simulink model "Full_system_3DOF"  (R2015b)
settings: Solver=ode45  StartTime=0.0  StopTime=55  FixedStep=0.0001  RelTol=eps
values from neighbouring files (symbols this model uses):
  All_Inertia = 1e-9*[177248429.51 3410266.03 17326.3 ... (first row only)    [init_sim_3DOF.m]    (also in init_sim_4DOF.m)
  B_m = 0.5*8815e-4    (= 0.44075)    [init_sim_3DOF.m]
  c_B = 0    [init_sim_1DOF.m]    (also in init_sim_4DOF.m)
  c_flux = 1    [init_sim_3DOF.m]
  c_G = 0.5    [init_sim_3DOF.m]    (also in init_sim_4DOF.m = 0)
  c_trans = c_G    (= 0.5)    [init_sim_3DOF.m]    (also in init_sim_4DOF.m = 0)
  Float_CoM = CoM-N_DCM_G*G_r_CB    [init_sim_3DOF.m]    (also in init_sim_4DOF.m = CoM+N_DCM_G*G_r_CB)
  Float_init_vel = OS_init_vel    [init_sim_3DOF.m]    (also in init_sim_4DOF.m)
  OS_init_omega = 0    [init_sim_1DOF.m]    (also in init_sim_3DOF.m; init_sim_4DOF.m = [0 0 0]'; init_sim_6DOF.m = [0 0 0]')
  OS_rotation = 0    [init_sim_1DOF.m]    (also in init_sim_3DOF.m; init_sim_4DOF.m = [0 0 0]'; init_sim_6DOF.m = [0 0 0]')
  SROA_Inertia = 1e7*eye(3)    [init_sim_3DOF.m]    (also in init_sim_4DOF.m)
  SROA_Mass = 100000    [init_sim_3DOF.m]    (also in init_sim_4DOF.m)
  V = [0 0 0 0 0 0]'    [init_sim_1DOF.m]    (also in init_sim_3DOF.m; init_sim_4DOF.m; init_sim_6DOF.m)
  Whole_Mass = 12.38866    [init_sim_3DOF.m]    (also in init_sim_4DOF.m)
undefined symbols (not defined in the file or in its folder): EM_mu, EM_xyz, origin, OS_mu_0, OS_xyz_0
libraries: my_ACS_library x1
settings Model: Creator=user  LastModifiedBy=user
settings DataIOCC: SaveFormat=Array
settings DebuggingCC: SolverPrmCheckMsg=warning
settings HardwareCC: ProdBitPerPointer=32  ProdLargestAtomicFloat=None  ProdIntDivRoundTo=Undefined  ProdEndianess=Unspecified  ProdWordSize=32  ProdHWDeviceType=32-bit Generic
settings GRTTargetCC: GeneratePreprocessorConditionals=Disable all
settings ConfigComp: CovModelRefEnable=Off  CovSFcnEnable=off

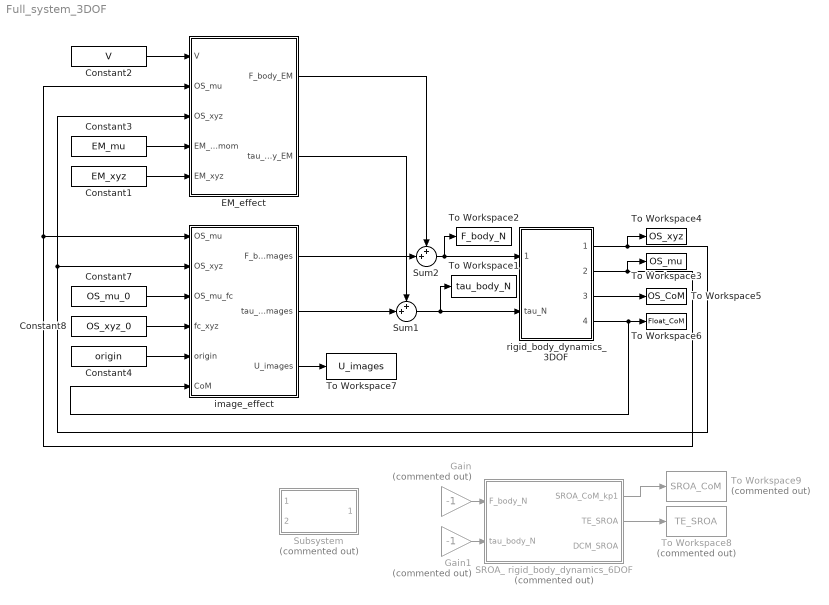
== system Full_system_3DOF ==
  Constant1 : Constant  Value=EM_xyz
  Constant2 : Constant  Value=V
  Constant3 : Constant  Value=EM_mu
  Constant4 : Constant  Value=origin
  Constant7 : Constant  Value=OS_mu_0  VectorParams1D=off
  Constant8 : Constant  Value=OS_xyz_0
  EM_effect : MATLAB Function  TreatAsAtomicUnit=on
  Gain : Gain  Commented=on  Gain=-1
  Gain1 : Gain  Commented=on  Gain=-1
  SROA_ rigid_body_dynamics_6DOF : Subsystem  Commented=on
  Subsystem : Subsystem  Commented=on
  Sum1 : Sum  Inputs=++|
  Sum2 : Sum  Inputs=++|
  To Workspace1 : ToWorkspace  VariableName=tau_body_N  SaveFormat=Timeseries  SampleTime=-1
  To Workspace2 : ToWorkspace  VariableName=F_body_N  SaveFormat=Timeseries  SampleTime=-1
  To Workspace3 : ToWorkspace  VariableName=OS_mu  SaveFormat=Timeseries  SampleTime=-1
  To Workspace4 : ToWorkspace  VariableName=OS_xyz  SaveFormat=Timeseries  SampleTime=-1
  To Workspace5 : ToWorkspace  VariableName=OS_CoM  SaveFormat=Timeseries  SampleTime=-1
  To Workspace6 : ToWorkspace  VariableName=Float_CoM  SaveFormat=Timeseries  SampleTime=-1
  To Workspace7 : ToWorkspace  VariableName=U_images  SaveFormat=Timeseries  SampleTime=-1
  To Workspace8 : ToWorkspace  Commented=on  VariableName=TE_SROA  SaveFormat=Timeseries  SampleTime=-1
  To Workspace9 : ToWorkspace  Commented=on  VariableName=SROA_CoM  SaveFormat=Timeseries  SampleTime=-1
  image_effect : MATLAB Function  TreatAsAtomicUnit=on
  rigid_body_dynamics_3DOF : Subsystem
  wires:
  Constant3/1 -> EM_effect/4(EM_magmom)
  Constant1/1 -> EM_effect/5(EM_xyz)
  image_effect/1(F_body_images) -> Sum2/2
  image_effect/2(tau_body_images) -> Sum1/2
  EM_effect/2(tau_body_EM) -> Sum1/1
  EM_effect/1(F_body_EM) -> Sum2/1
  image_effect/3(U_images) -> To Workspace7/1
  Sum2/1 -> To Workspace2/1, rigid_body_dynamics_3DOF/1(Force_N)
  Sum1/1 -> To Workspace1/1, rigid_body_dynamics_3DOF/2(tau_N)
  rigid_body_dynamics_3DOF/4(Float_CoM) -> image_effect/6(CoM), To Workspace6/1
  Constant2/1 -> EM_effect/1(V)
  rigid_body_dynamics_3DOF/1(OS_xyz) -> To Workspace4/1, EM_effect/3(OS_xyz), image_effect/2(OS_xyz)
  rigid_body_dynamics_3DOF/2(OS_mu) -> To Workspace3/1, EM_effect/2(OS_mu), image_effect/1(OS_mu)
  rigid_body_dynamics_3DOF/3(OS_CoM) -> To Workspace5/1
  Constant7/1 -> image_effect/3(OS_mu_fc)
  Constant8/1 -> image_effect/4(fc_xyz)
  Constant4/1 -> image_effect/5(origin)
  Gain/1 -> SROA_ rigid_body_dynamics_6DOF/1(F_body_N)
  Gain1/1 -> SROA_ rigid_body_dynamics_6DOF/2(tau_body_N)
  SROA_ rigid_body_dynamics_6DOF/2(TE_SROA) -> To Workspace8/1
  SROA_ rigid_body_dynamics_6DOF/1(SROA_CoM_kp1) -> To Workspace9/1

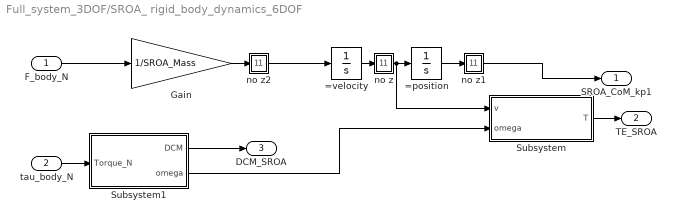
== system Full_system_3DOF/SROA_ rigid_body_dynamics_6DOF ==
  F_body_N : Inport
  tau_body_N : Inport  Port=2
  =position : Integrator  InitialCondition=[0 0 0]'
  =velocity : Integrator  InitialCondition=[0 0 0]'
  Gain : Gain  Gain=1/SROA_Mass
  Subsystem : Subsystem
  Subsystem1 : Subsystem
  no z : Subsystem
  no z1 : Subsystem
  no z2 : Subsystem
  SROA_CoM_kp1 : Outport
  TE_SROA : Outport  Port=2  PortDimensions=1
  DCM_SROA : Outport  Port=3  PortDimensions=[3 3]
  wires:
  Subsystem/1(T) -> TE_SROA/1
  F_body_N/1 -> Gain/1
  =velocity/1 -> no z/1(In1)
  no z/1(Out1) -> Subsystem/1(v), =position/1
  =position/1 -> no z1/1(In1)
  Gain/1 -> no z2/1(In1)
  no z2/1(Out1) -> =velocity/1
  no z1/1(Out1) -> SROA_CoM_kp1/1
  tau_body_N/1 -> Subsystem1/1(Torque_N)
  Subsystem1/2(omega) -> Subsystem/2(omega)
  Subsystem1/1(DCM) -> DCM_SROA/1

== system Full_system_3DOF/Subsystem ==
  SROA_CoM : Inport
  SROA_DCM : Inport  Port=2
  Constant2 : Constant  Value=origin
  MATLAB Function : MATLAB Function  TreatAsAtomicUnit=on
  SROA_origin : Outport
  wires:
  Constant2/1 -> MATLAB Function/1(origin)
  SROA_CoM/1 -> MATLAB Function/2(CoM)
  MATLAB Function/1(origin_new) -> SROA_origin/1
  SROA_DCM/1 -> MATLAB Function/3(DCM)

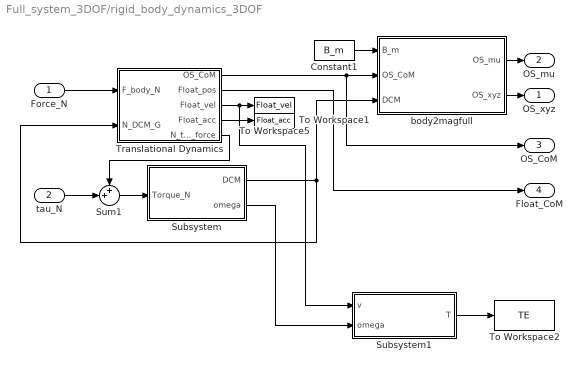
== system Full_system_3DOF/rigid_body_dynamics_3DOF ==
  Force_N : Inport
  tau_N : Inport  Port=2
  Constant1 : Constant  Value=B_m
  Subsystem : Subsystem
  Subsystem1 : Subsystem
  Sum1 : Sum  Inputs=++|
  To Workspace1 : ToWorkspace  VariableName=Float_acc  SaveFormat=Timeseries  SampleTime=-1
  To Workspace2 : ToWorkspace  VariableName=TE  SaveFormat=Timeseries  SampleTime=-1
  To Workspace5 : ToWorkspace  VariableName=Float_vel  SaveFormat=Timeseries  SampleTime=-1
  Translational Dynamics : Subsystem
  body2magfull : MATLAB Function  TreatAsAtomicUnit=on
  OS_xyz : Outport
  OS_mu : Outport  Port=2
  OS_CoM : Outport  Port=3
  Float_CoM : Outport  Port=4
  wires:
  Force_N/1 -> Translational Dynamics/1(F_body_N)
  tau_N/1 -> Sum1/2
  body2magfull/2(OS_xyz) -> OS_xyz/1
  body2magfull/1(OS_mu) -> OS_mu/1
  Translational Dynamics/1(OS_CoM) -> OS_CoM/1, body2magfull/2(OS_CoM)
  Translational Dynamics/2(Float_pos) -> Float_CoM/1
  Sum1/1 -> Subsystem/1(Torque_N)
  Subsystem/1(DCM) -> body2magfull/3(DCM), Translational Dynamics/2(N_DCM_G)
  Translational Dynamics/3(Float_vel) -> Subsystem1/1(v), To Workspace5/1
  Translational Dynamics/4(Float_acc) -> To Workspace1/1
  Subsystem1/1(T) -> To Workspace2/1
  Subsystem/2(omega) -> Subsystem1/2(omega)
  Translational Dynamics/5(N_tau_force) -> Sum1/1
  Constant1/1 -> body2magfull/1(B_m)

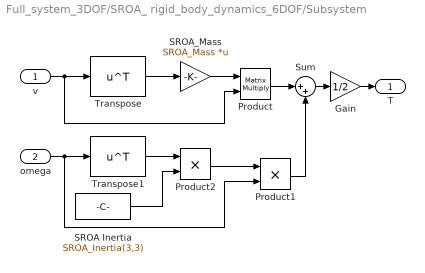
== system Full_system_3DOF/SROA_ rigid_body_dynamics_6DOF/Subsystem ==
  v : Inport
  omega : Inport  Port=2
  Gain : Gain  Gain=1/2
  Product : Product  Multiplication=Matrix(*)
  Product1 : Product
  Product2 : Product
  SROA Inertia : Constant  Value=SROA_Inertia(3,3)
  SROA_Mass : Gain  Gain=SROA_Mass  Multiplication=Matrix(K*u)
  Sum : Sum  Inputs=|++
  Transpose : Math  Operator=transpose  SaturateOnIntegerOverflow=on
  Transpose1 : Math  Operator=transpose  SaturateOnIntegerOverflow=on
  T : Outport
  wires:
  v/1 -> Product/2, Transpose/1
  Transpose/1 -> SROA_Mass/1
  SROA_Mass/1 -> Product/1
  Sum/1 -> Gain/1
  Gain/1 -> T/1
  omega/1 -> Product1/2, Transpose1/1
  Transpose1/1 -> Product2/1
  Product2/1 -> Product1/1
  Product/1 -> Sum/1
  Product1/1 -> Sum/2
  SROA Inertia/1 -> Product2/2

== system Full_system_3DOF/SROA_ rigid_body_dynamics_6DOF/Subsystem1 ==
  Torque_N : Inport
  Constant1 : Constant  Value=[0 0 1]'
  Subsystem : Subsystem
  ea2DCM : my_ACS_library/attitude conversions/ea2DCM
  DCM : Outport
  omega : Outport  Port=2
  wires:
  Constant1/1 -> Subsystem/2(a_hat), ea2DCM/2
  ea2DCM/1 -> DCM/1
  Torque_N/1 -> Subsystem/1(tau)
  Subsystem/1(phi) -> ea2DCM/1
  Subsystem/2(omega) -> omega/1

== system Full_system_3DOF/SROA_ rigid_body_dynamics_6DOF/no z ==
  In1 : Inport
  Demux : Demux  Outputs=3
  Ground : Ground
  Mux : Mux  Inputs=3
  Terminator : Terminator
  Out1 : Outport  PortDimensions=3
  wires:
  Demux/2 -> Mux/2
  In1/1 -> Demux/1
  Ground/1 -> Mux/3
  Demux/3 -> Terminator/1
  Demux/1 -> Mux/1
  Mux/1 -> Out1/1

== system Full_system_3DOF/SROA_ rigid_body_dynamics_6DOF/no z1 ==
  In1 : Inport
  Demux : Demux  Outputs=3
  Ground : Ground
  Mux : Mux  Inputs=3
  Terminator : Terminator
  Out1 : Outport  PortDimensions=3
  wires:
  Demux/2 -> Mux/2
  In1/1 -> Demux/1
  Ground/1 -> Mux/3
  Demux/3 -> Terminator/1
  Demux/1 -> Mux/1
  Mux/1 -> Out1/1

== system Full_system_3DOF/SROA_ rigid_body_dynamics_6DOF/no z2 ==
  In1 : Inport
  Demux : Demux  Outputs=3
  Ground : Ground
  Mux : Mux  Inputs=3
  Terminator : Terminator
  Out1 : Outport  PortDimensions=3
  wires:
  Demux/2 -> Mux/2
  In1/1 -> Demux/1
  Ground/1 -> Mux/3
  Demux/3 -> Terminator/1
  Demux/1 -> Mux/1
  Mux/1 -> Out1/1

== system Full_system_3DOF/rigid_body_dynamics_3DOF/Subsystem ==
  Torque_N : Inport
  Constant1 : Constant  Value=[0 0 1]'
  Subsystem : Subsystem
  ea2DCM : Subsystem
  DCM : Outport
  omega : Outport  Port=2
  wires:
  Constant1/1 -> Subsystem/2(a_hat), ea2DCM/2(axis)
  ea2DCM/1(DCM) -> DCM/1
  Torque_N/1 -> Subsystem/1(tau)
  Subsystem/1(phi) -> ea2DCM/1(angle)
  Subsystem/2(omega) -> omega/1

== system Full_system_3DOF/rigid_body_dynamics_3DOF/Subsystem1 ==
  v : Inport
  omega : Inport  Port=2
  Constant : Constant  Value=All_Inertia(3,3)
  Gain : Gain  Gain=1/2
  Gain1 : Gain  Gain=Whole_Mass  Multiplication=Matrix(K*u)
  Product : Product  Multiplication=Matrix(*)
  Product1 : Product
  Product2 : Product
  Sum : Sum  Inputs=|++
  Transpose : Math  Operator=transpose  SaturateOnIntegerOverflow=on
  T : Outport  PortDimensions=1
  wires:
  v/1 -> Product/2, Transpose/1
  Transpose/1 -> Gain1/1
  Gain1/1 -> Product/1
  Sum/1 -> Gain/1
  Gain/1 -> T/1
  omega/1 -> Product2/1, Product1/2
  Product2/1 -> Product1/1
  Product/1 -> Sum/1
  Product1/1 -> Sum/2
  Constant/1 -> Product2/2

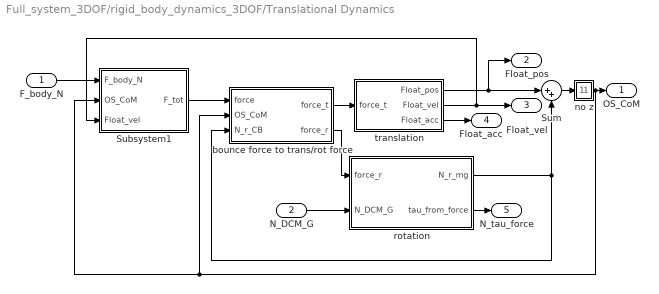
== system Full_system_3DOF/rigid_body_dynamics_3DOF/Translational Dynamics ==
  F_body_N : Inport
  N_DCM_G : Inport  Port=2
  Subsystem1 : Subsystem
  Sum : Sum  Inputs=|++
  bounce force to trans/rot force : Subsystem
  no z : Subsystem
  rotation : Subsystem
  translation : Subsystem
  OS_CoM : Outport
  Float_pos : Outport  Port=2
  Float_vel : Outport  Port=3
  Float_acc : Outport  Port=4
  N_tau_force : Outport  Port=5
  wires:
  rotation/2(tau_from_force) -> N_tau_force/1
  F_body_N/1 -> Subsystem1/1(F_body_N)
  bounce force to trans/rot force/1(force_t) -> translation/1(force_t)
  translation/1(Float_pos) -> Sum/1, Float_pos/1
  bounce force to trans/rot force/2(force_r) -> rotation/1(force_r)
  rotation/1(N_r_mg) -> Sum/2, bounce force to trans/rot force/3(N_r_CB)
  Subsystem1/1(F_tot) -> bounce force to trans/rot force/1(force)
  N_DCM_G/1 -> rotation/2(N_DCM_G)
  translation/2(Float_vel) -> Float_vel/1, Subsystem1/3(Float_vel)
  translation/3(Float_acc) -> Float_acc/1
  Sum/1 -> no z/1(In1)
  no z/1(Out1) -> Subsystem1/2(OS_CoM), bounce force to trans/rot force/2(OS_CoM), OS_CoM/1

== system Full_system_3DOF/SROA_ rigid_body_dynamics_6DOF/Subsystem1/Subsystem ==
  note: tau
  tau : Inport
  a_hat : Inport  Port=2
  Dot Product : DotProduct  InputSameDT=on  OutDataTypeStr=Inherit: Inherit via internal rule
  Gain : Gain  Gain=1/SROA_Inertia(3,3)
  Gain1 : Gain  Gain=c_B
  Sum : Sum  Inputs=|+-
  int dw : Integrator
  int w : Integrator
  phi : Outport
  omega : Outport  Port=2
  wires:
  a_hat/1 -> Dot Product/2
  Gain/1 -> int dw/1  "dw"
  int dw/1 -> omega/1, Gain1/1, int w/1  "w"
  int w/1 -> phi/1  "phi"
  tau/1 -> Dot Product/1
  Sum/1 -> Gain/1
  Dot Product/1 -> Sum/1
  Gain1/1 -> Sum/2

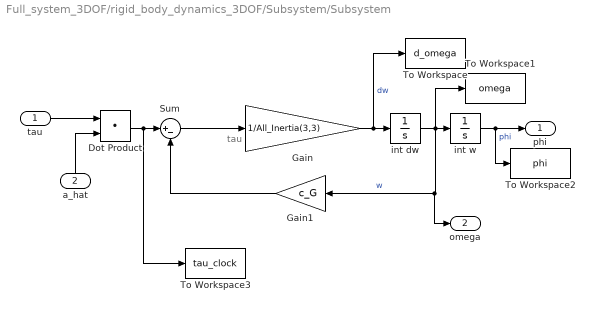
== system Full_system_3DOF/rigid_body_dynamics_3DOF/Subsystem/Subsystem ==
  note: tau
  tau : Inport
  a_hat : Inport  Port=2
  Dot Product : DotProduct  InputSameDT=on  OutDataTypeStr=Inherit: Inherit via internal rule
  Gain : Gain  Gain=1/All_Inertia(3,3)
  Gain1 : Gain  Gain=c_G
  Sum : Sum  Inputs=|+-
  To Workspace : ToWorkspace  VariableName=d_omega  SaveFormat=Timeseries  SampleTime=-1
  To Workspace1 : ToWorkspace  VariableName=omega  SaveFormat=Timeseries  SampleTime=-1
  To Workspace2 : ToWorkspace  VariableName=phi  SaveFormat=Timeseries  SampleTime=-1
  To Workspace3 : ToWorkspace  VariableName=tau_clock  SaveFormat=Timeseries  SampleTime=-1
  int dw : Integrator  InitialCondition=OS_init_omega
  int w : Integrator  InitialCondition=OS_rotation
  phi : Outport
  omega : Outport  Port=2
  wires:
  a_hat/1 -> Dot Product/2
  Gain/1 -> To Workspace/1, int dw/1  "dw"
  int dw/1 -> omega/1, Gain1/1, To Workspace1/1, int w/1  "w"
  int w/1 -> To Workspace2/1, phi/1  "phi"
  tau/1 -> Dot Product/1
  Sum/1 -> Gain/1
  Dot Product/1 -> To Workspace3/1, Sum/1
  Gain1/1 -> Sum/2

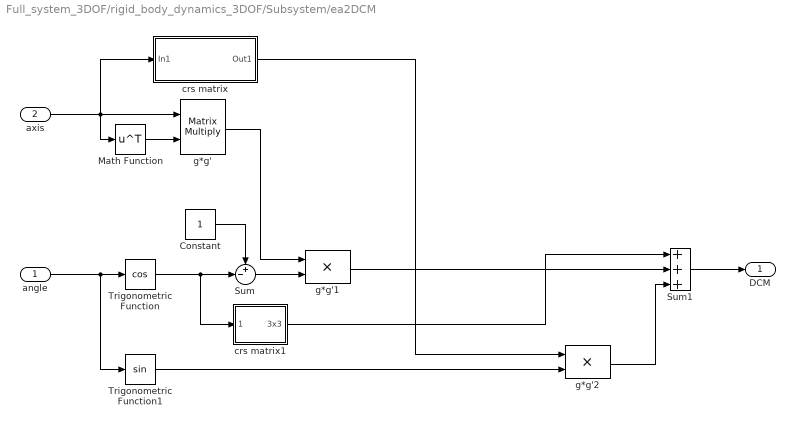
== system Full_system_3DOF/rigid_body_dynamics_3DOF/Subsystem/ea2DCM ==
  angle : Inport
  axis : Inport  Port=2
  Constant : Constant
  Math Function : Math  Operator=transpose  SaturateOnIntegerOverflow=on
  Sum : Sum  Inputs=+-|  SaturateOnIntegerOverflow=on
  Sum1 : Sum  Inputs=+++  SaturateOnIntegerOverflow=on
  Trigonometric Function : Trigonometry  Operator=cos
  Trigonometric Function1 : Trigonometry
  crs matrix : Subsystem
  crs matrix1 : Subsystem
  g*g' : Product  Multiplication=Matrix(*)  SaturateOnIntegerOverflow=on  OutDataTypeStr=Inherit: Same as first input
  g*g'1 : Product  SaturateOnIntegerOverflow=on  OutDataTypeStr=Inherit: Same as first input
  g*g'2 : Product  SaturateOnIntegerOverflow=on  OutDataTypeStr=Inherit: Same as first input
  DCM : Outport
  wires:
  g*g'2/1 -> Sum1/3
  crs matrix1/1(3x3) -> Sum1/1
  Sum1/1 -> DCM/1
  crs matrix/1(Out1) -> g*g'2/1
  Trigonometric Function1/1 -> g*g'2/2
  g*g'1/1 -> Sum1/2
  g*g'/1 -> g*g'1/1
  Math Function/1 -> g*g'/2
  axis/1 -> crs matrix/1(In1), Math Function/1, g*g'/1
  Sum/1 -> g*g'1/2
  Constant/1 -> Sum/1
  Trigonometric Function/1 -> crs matrix1/1(make), Sum/2
  angle/1 -> Trigonometric Function1/1, Trigonometric Function/1

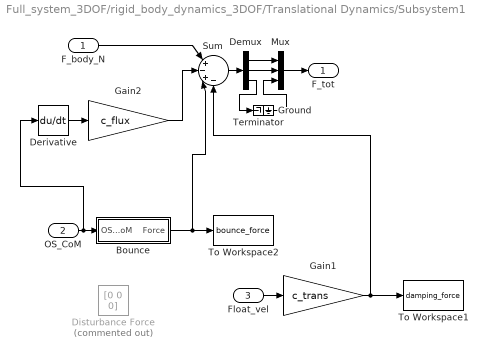
== system Full_system_3DOF/rigid_body_dynamics_3DOF/Translational Dynamics/Subsystem1 ==
  F_body_N : Inport
  OS_CoM : Inport  Port=2
  Float_vel : Inport  Port=3
  Bounce : Subsystem
  Demux : Demux  Outputs=3
  Derivative : Derivative
  Disturbance Force : Constant  Commented=on  Value=[0 0 0]
  Gain1 : Gain  Gain=c_trans
  Gain2 : Gain  Gain=c_flux
  Ground : Ground
  Mux : Mux  Inputs=3
  Sum : Sum  Inputs=|+-+-
  Terminator : Terminator
  To Workspace1 : ToWorkspace  VariableName=damping_force  SaveFormat=Timeseries  SampleTime=-1
  To Workspace2 : ToWorkspace  VariableName=bounce_force  SaveFormat=Timeseries  SampleTime=-1
  F_tot : Outport
  wires:
  Sum/1 -> Demux/1
  Ground/1 -> Mux/3
  Demux/3 -> Terminator/1
  Demux/2 -> Mux/2
  Demux/1 -> Mux/1
  Mux/1 -> F_tot/1
  Gain2/1 -> Sum/2
  F_body_N/1 -> Sum/1
  Gain1/1 -> To Workspace1/1, Sum/4
  Bounce/1(Force) -> To Workspace2/1, Sum/3
  OS_CoM/1 -> Derivative/1, Bounce/1(OS_CoM)
  Float_vel/1 -> Gain1/1
  Derivative/1 -> Gain2/1

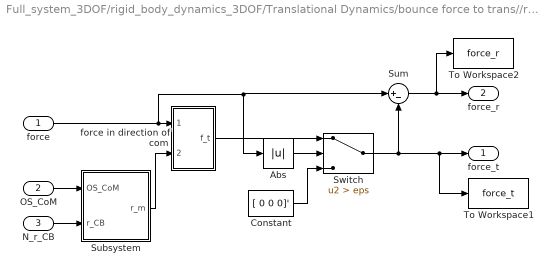
== system Full_system_3DOF/rigid_body_dynamics_3DOF/Translational Dynamics/bounce force to trans//rot force ==
  force : Inport
  OS_CoM : Inport  Port=2
  N_r_CB : Inport  Port=3
  Abs : Abs
  Constant : Constant  Value=[ 0 0 0]'
  Subsystem : Subsystem
  Sum : Sum  Inputs=|+-
  Switch : Switch  Criteria=u2 > Threshold  Threshold=eps
  To Workspace1 : ToWorkspace  VariableName=force_t  SaveFormat=Timeseries  SampleTime=-1
  To Workspace2 : ToWorkspace  VariableName=force_r  SaveFormat=Timeseries  SampleTime=-1
  force in direction of com : Subsystem
  force_t : Outport
  force_r : Outport  Port=2
  wires:
  OS_CoM/1 -> Subsystem/1(OS_CoM)
  N_r_CB/1 -> Subsystem/2(r_CB)
  Subsystem/1(r_m) -> force in direction of com/2(r_m)
  force/1 -> Abs/1, Sum/1, force in direction of com/1(force)
  Switch/1 -> Sum/2, To Workspace1/1, force_t/1
  force in direction of com/1(f_t) -> Switch/1
  Constant/1 -> Switch/3
  Sum/1 -> force_r/1, To Workspace2/1
  Abs/1 -> Switch/2

== system Full_system_3DOF/rigid_body_dynamics_3DOF/Translational Dynamics/no z ==
  In1 : Inport
  Demux : Demux  Outputs=3
  Ground : Ground
  Mux : Mux  Inputs=3
  Terminator : Terminator
  Out1 : Outport
  wires:
  Demux/2 -> Mux/2
  In1/1 -> Demux/1
  Ground/1 -> Mux/3
  Demux/3 -> Terminator/1
  Demux/1 -> Mux/1
  Mux/1 -> Out1/1

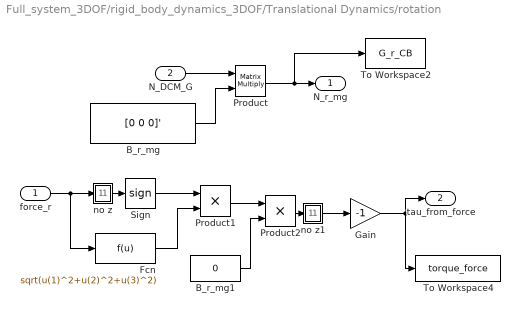
== system Full_system_3DOF/rigid_body_dynamics_3DOF/Translational Dynamics/rotation ==
  force_r : Inport
  N_DCM_G : Inport  Port=2
  B_r_mg : Constant  Value=[0 0 0]'
  B_r_mg1 : Constant  Value=0
  Fcn : Fcn  Expr=sqrt(u(1)^2+u(2)^2+u(3)^2)
  Gain : Gain  Gain=-1
  Product : Product  Multiplication=Matrix(*)
  Product1 : Product
  Product2 : Product
  Sign : Signum
  To Workspace2 : ToWorkspace  VariableName=G_r_CB  SaveFormat=Timeseries  SampleTime=-1
  To Workspace4 : ToWorkspace  VariableName=torque_force  SaveFormat=Timeseries  SampleTime=-1
  no z : Subsystem
  no z1 : Subsystem
  N_r_mg : Outport  PortDimensions=3
  tau_from_force : Outport  Port=2
  wires:
  B_r_mg/1 -> Product/2
  Product/1 -> To Workspace2/1, N_r_mg/1
  N_DCM_G/1 -> Product/1
  force_r/1 -> no z/1(In1), Fcn/1
  no z/1(Out1) -> Sign/1
  Sign/1 -> Product1/1
  Fcn/1 -> Product1/2
  Product1/1 -> Product2/1
  B_r_mg1/1 -> Product2/2
  Product2/1 -> no z1/1(In1)
  no z1/1(Out1) -> Gain/1
  Gain/1 -> tau_from_force/1, To Workspace4/1

== system Full_system_3DOF/rigid_body_dynamics_3DOF/Translational Dynamics/translation ==
  force_t : Inport
  =position : Integrator  InitialCondition=Float_CoM
  =velocity : Integrator  InitialCondition=Float_init_vel
  Gain : Gain  Gain=1/Whole_Mass
  Scope : Scope
  no z : Subsystem
  no z1 : Subsystem
  no z2 : Subsystem
  Float_pos : Outport  PortDimensions=3
  Float_vel : Outport  Port=2  PortDimensions=3
  Float_acc : Outport  Port=3  PortDimensions=3
  wires:
  force_t/1 -> Gain/1
  =velocity/1 -> no z/1(In1)
  no z/1(Out1) -> Float_vel/1, =position/1
  =position/1 -> no z1/1(In1)
  no z1/1(Out1) -> Float_pos/1, Scope/1
  Gain/1 -> no z2/1(In1)
  no z2/1(Out1) -> Float_acc/1, =velocity/1

== system Full_system_3DOF/rigid_body_dynamics_3DOF/Subsystem/ea2DCM/crs matrix ==
  In1 : Inport
  Constant : Constant  Value=0
  Demux : Demux  Outputs=3
  Gain : Gain  Gain=-1  SaturateOnIntegerOverflow=on  OutDataTypeStr=Inherit: Same as input  ParamDataTypeStr=Inherit: Same as input
  Gain1 : Gain  Gain=-1  SaturateOnIntegerOverflow=on  OutDataTypeStr=Inherit: Same as input  ParamDataTypeStr=Inherit: Same as input
  Gain2 : Gain  Gain=-1  SaturateOnIntegerOverflow=on  OutDataTypeStr=Inherit: Same as input  ParamDataTypeStr=Inherit: Same as input
  Matrix Concatenation : Concatenate  NumInputs=3  Mode=Multidimensional array  ConcatenateDimension=2
  Mux : Mux  Inputs=3
  Mux1 : Mux  Inputs=3
  Mux2 : Mux  Inputs=3
  Out1 : Outport
  wires:
  Matrix Concatenation/1 -> Out1/1
  Gain2/1 -> Mux2/2
  Mux2/1 -> Matrix Concatenation/3
  Mux1/1 -> Matrix Concatenation/2
  Demux/1 -> Gain2/1, Mux1/3
  Gain1/1 -> Mux1/1
  Mux/1 -> Matrix Concatenation/1
  Gain/1 -> Mux/3
  Demux/2 -> Mux2/1, Gain/1
  Demux/3 -> Gain1/1, Mux/2
  Constant/1 -> Mux2/3, Mux/1, Mux1/2
  In1/1 -> Demux/1

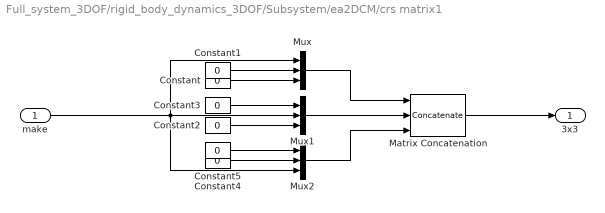
== system Full_system_3DOF/rigid_body_dynamics_3DOF/Subsystem/ea2DCM/crs matrix1 ==
  make : Inport
  Constant{,1..5} (6 alike) : Constant  Value=0
  Matrix Concatenation : Concatenate  NumInputs=3  Mode=Multidimensional array  ConcatenateDimension=2
  Mux : Mux  Inputs=3
  Mux1 : Mux  Inputs=3
  Mux2 : Mux  Inputs=3
  3x3 : Outport
  wires:
  Constant5/1 -> Mux2/1
  Constant4/1 -> Mux2/2
  Constant3/1 -> Mux1/1
  Constant2/1 -> Mux1/3
  Constant1/1 -> Mux/2
  Constant/1 -> Mux/3
  Matrix Concatenation/1 -> 3x3/1
  Mux2/1 -> Matrix Concatenation/3
  Mux1/1 -> Matrix Concatenation/2
  Mux/1 -> Matrix Concatenation/1
  make/1 -> Mux2/3, Mux1/2, Mux/1

== system Full_system_3DOF/rigid_body_dynamics_3DOF/Translational Dynamics/Subsystem1/Bounce ==
  OS_CoM : Inport
  Gain : Gain  Gain=-1
  Product : Product
  Saturation : Saturate  Commented=on  UpperLimit=100  LowerLimit=-100
  Subsystem : Subsystem
  Force : Outport
  wires:
  Gain/1 -> Saturation/1
  Product/1 -> Gain/1
  Subsystem/1(k(x)) -> Product/1
  OS_CoM/1 -> Subsystem/1(OS_CoM), Product/2
  Saturation/1 -> Force/1

== system Full_system_3DOF/rigid_body_dynamics_3DOF/Translational Dynamics/bounce force to trans//rot force/Subsystem ==
  OS_CoM : Inport
  r_CB : Inport  Port=2
  Constant : Constant  Value=0.1
  Product : Product
  Product1 : Product
  Sum : Sum  Inputs=|++
  norm3x1 : Fcn  Expr=sqrt(u(1)^2+u(2)^2+u(3)^2)
  r_m : Outport
  wires:
  r_CB/1 -> Sum/2
  OS_CoM/1 -> Product/2, norm3x1/1
  norm3x1/1 -> Product/1
  Product/1 -> Product1/1
  Constant/1 -> Product1/2
  Sum/1 -> r_m/1  "r_m"
  Product1/1 -> Sum/1  "r_g"

== system Full_system_3DOF/rigid_body_dynamics_3DOF/Translational Dynamics/bounce force to trans//rot force/force in direction of com ==
  force : Inport
  r_m : Inport  Port=2
  Divide : Product  Inputs=*/
  Gain : Gain  Gain=-1
  Product : Product
  Product1 : Product
  Trigonometric Function : Trigonometry  Operator=cos
  angle b2n vec : Subsystem
  norm3x1 : Fcn  Expr=sqrt(u(1)^2+u(2)^2+u(3)^2)
  norm3x1.2 : Fcn  Expr=sqrt(u(1)^2+u(2)^2+u(3)^2)
  f_t : Outport
  wires:
  norm3x1.2/1 -> Divide/2
  Trigonometric Function/1 -> Product/2
  Divide/1 -> Product1/2  "r_hat"
  force/1 -> norm3x1/1, angle b2n vec/1(u)
  Gain/1 -> Divide/1, angle b2n vec/2(v)
  r_m/1 -> norm3x1.2/1, Gain/1
  Product1/1 -> f_t/1
  angle b2n vec/1(theta) -> Trigonometric Function/1
  Product/1 -> Product1/1
  norm3x1/1 -> Product/1

== system Full_system_3DOF/rigid_body_dynamics_3DOF/Translational Dynamics/rotation/no z ==
  In1 : Inport
  Demux : Demux  Outputs=3
  Terminator : Terminator
  Terminator1 : Terminator
  Out1 : Outport
  wires:
  In1/1 -> Demux/1
  Demux/3 -> Terminator/1
  Demux/2 -> Terminator1/1
  Demux/1 -> Out1/1

== system Full_system_3DOF/rigid_body_dynamics_3DOF/Translational Dynamics/rotation/no z1 ==
  In1 : Inport
  Ground : Ground
  Ground1 : Ground
  Mux : Mux  Inputs=3
  Out1 : Outport
  wires:
  Mux/1 -> Out1/1
  In1/1 -> Mux/3
  Ground/1 -> Mux/1
  Ground1/1 -> Mux/2

== system Full_system_3DOF/rigid_body_dynamics_3DOF/Translational Dynamics/translation/no z ==
  In1 : Inport
  Demux : Demux  Outputs=3
  Ground : Ground
  Mux : Mux  Inputs=3
  Terminator : Terminator
  Out1 : Outport  PortDimensions=3
  wires:
  Demux/2 -> Mux/2
  In1/1 -> Demux/1
  Ground/1 -> Mux/3
  Demux/3 -> Terminator/1
  Demux/1 -> Mux/1
  Mux/1 -> Out1/1

== system Full_system_3DOF/rigid_body_dynamics_3DOF/Translational Dynamics/translation/no z1 ==
  In1 : Inport
  Demux : Demux  Outputs=3
  Ground : Ground
  Mux : Mux  Inputs=3
  Terminator : Terminator
  Out1 : Outport  PortDimensions=3
  wires:
  Demux/2 -> Mux/2
  In1/1 -> Demux/1
  Ground/1 -> Mux/3
  Demux/3 -> Terminator/1
  Demux/1 -> Mux/1
  Mux/1 -> Out1/1

== system Full_system_3DOF/rigid_body_dynamics_3DOF/Translational Dynamics/translation/no z2 ==
  In1 : Inport
  Demux : Demux  Outputs=3
  Ground : Ground
  Mux : Mux  Inputs=3
  Terminator : Terminator
  Out1 : Outport  PortDimensions=3
  wires:
  Demux/2 -> Mux/2
  In1/1 -> Demux/1
  Ground/1 -> Mux/3
  Demux/3 -> Terminator/1
  Demux/1 -> Mux/1
  Mux/1 -> Out1/1

== system Full_system_3DOF/rigid_body_dynamics_3DOF/Translational Dynamics/Subsystem1/Bounce/Subsystem ==
  OS_CoM : Inport
  Display : Display
  Fcn : Fcn  Expr=10*exp(10000*u)
  Subsystem : Subsystem
  k(x) : Outport
  wires:
  Fcn/1 -> k(x)/1
  Subsystem/1(x) -> Fcn/1, Display/1
  OS_CoM/1 -> Subsystem/1(OS_CoM)

== system Full_system_3DOF/rigid_body_dynamics_3DOF/Translational Dynamics/bounce force to trans//rot force/force in direction of com/angle b2n vec ==
  u : Inport
  v : Inport  Port=2
  Display : Display
  Divide : Product  Inputs=*/
  Divide1 : Product  Inputs=/*
  Dot Product : DotProduct  InputSameDT=on  OutDataTypeStr=Inherit: Inherit via internal rule
  Trigonometric Function : Trigonometry  Operator=acos
  norm3x1 : Fcn  Expr=sqrt(u(1)^2+u(2)^2+u(3)^2)
  norm3x1.2 : Fcn  Expr=sqrt(u(1)^2+u(2)^2+u(3)^2)
  theta : Outport
  wires:
  Trigonometric Function/1 -> theta/1
  Divide1/1 -> Trigonometric Function/1
  norm3x1/1 -> Display/1, Divide1/1
  Divide/1 -> Divide1/2
  norm3x1.2/1 -> Divide/2
  Dot Product/1 -> Divide/1
  v/1 -> norm3x1.2/1, Dot Product/2
  u/1 -> norm3x1/1, Dot Product/1

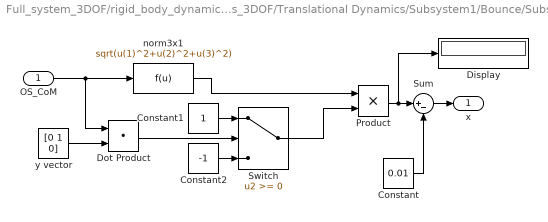
== system Full_system_3DOF/rigid_body_dynamics_3DOF/Translational Dynamics/Subsystem1/Bounce/Subsystem/Subsystem ==
  OS_CoM : Inport
  Constant : Constant  Value=0.01
  Constant1 : Constant
  Constant2 : Constant  Value=-1
  Display : Display
  Dot Product : DotProduct  InputSameDT=on  OutDataTypeStr=Inherit: Inherit via internal rule
  Product : Product
  Sum : Sum  Inputs=|+-
  Switch : Switch
  norm3x1 : Fcn  Expr=sqrt(u(1)^2+u(2)^2+u(3)^2)
  y vector : Constant  Value=[0 1 0]
  x : Outport
  wires:
  Switch/1 -> Product/2
  Constant2/1 -> Switch/3
  Constant1/1 -> Switch/1
  Product/1 -> Sum/1, Display/1
  Sum/1 -> x/1
  Constant/1 -> Sum/2
  Dot Product/1 -> Switch/2
  OS_CoM/1 -> Dot Product/1, norm3x1/1
  norm3x1/1 -> Product/1
  y vector/1 -> Dot Product/2

== matlab function Full_system_3DOF/EM_effect ==
  data: V input; OS_mu input; F_body_EM output; OS_xyz input; EM_magmom input; EM_xyz input; tau_body_EM output
function [F_body_EM,tau_body_EM]=EM_effect(V,OS_mu,OS_xyz,EM_magmom,EM_xyz)
%% Calculate the needed electromagnet voltage with a pseudoinverse
    %initialize a placeholder for the pseudoinverse
    A=zeros(6,length(V));
    
    %sift through all the electromagnets to back out portion of force
    %and torque generated from each individually
    for i=1:length(V) 
        %initialize sum of electromagnet contribution acting on each
        %permanent magnet due to electromagnet i
        dF_tot=zeros(1,3); 
        dtau_tot=zeros(1,3);
        %calculate electromagnet affect on force and torque on body through
        %all the permanent magnets
        for j=1:size(OS_xyz,1) 
            %in this case, the magnetic moment dipole being acted on is the 
            %permanent magnet, following Villani convention
            mu_mag_i=OS_mu(j,:);
            pos_mag_i=OS_xyz(j,:);
            %the magnetic moment dipole acting on magnet i is the
            %electromagnet
            mu_mag_j=EM_magmom(i,:);
            pos_mag_j=EM_xyz(i,:);
            %calculate_dV is a variation of villani. Villani requires mu
            %components and the position vector between them. Within
            %calculate_dV, the electromagnet's magnetic dipole/voltage is
            %substituted for force and torque per unit Volt
            [dF_dV,dtau_dV]=calculate_dV(mu_mag_i,pos_mag_i,mu_mag_j,pos_mag_j);
            %sum over each permanent magnet
            dF_tot=dF_tot+dF_dV;
            dtau_tot=dtau_tot+dtau_dV;
        end
        %fill in the portion of the pseudoinverse needed to calculate
        %electromagnetic contribution
        A(:,i)=[dF_tot';dtau_tot'];
    end
    %voltage calculated for this time step using the pseudoinverse
    y=A*V;
    F_body_EM=y(1:3);
    tau_body_EM=y(4:6);
end
    
function [dF_dV,dtau_dV]=calculate_dV(mu_mag_i,pos_mag_i,mu_mag_j,pos_mag_j)
%this function calculates force and torque per voltage acting on the 
%source magnet from an electromagnet
%mu_mag_i is the magnetic moment dipole of a magnet i
%mu_mag_j is the magnetic moment dipole of the electromagnet
%pos_mag_i is the position of the magnet i
%pos_mag_j is the position of the electromagnet

%the following parameters follow Laura's past experiments
%area enclosed by the electromagnet's current loop
A=0.001829214; %m^2
%number of turns in the electromagnet
T=1060;
%resistance of electromagnet
R=16.8; %Ohmsa
%the permeability of free space, mu_0
mu_0=4*pi*10^-7; %N/A^2

%the following parameters are required by Villani's analytical equations
%for forces and torques on two magnetic dipoles
rho_mji=pos_mag_j-pos_mag_i;
mu_mj_dV=A*T/R*mu_mag_j;
%the voltage is directly proportional to the force and torque applied on
%the magnetic dipole, making the calculation linear and relatively easy

[dF_dV,dtau_dV]=villani(mu_0,mu_mj_dV,mu_mag_i,rho_mji);
%the dF_dV dtau_dV will be evaluated for each electromagnet
%where [F; tau]=[dF_dV;dtau_dV]*[V] 
%V is a 6x1 column vector consisting of V_n for electromagnet n
%F is a 3x1 column vector consisting of forces in the x, y, and z
%tau is a 3x1 column vector consisting of torques in the x, y, and z
%[dF_dV;dtau_dV] is a 6x6 matrix consisting of the contribution of force
%and torque per volt from each electromagnet

end

== matlab function Full_system_3DOF/Subsystem/MATLAB Function ==
  data: origin input; origin_new output; CoM input; DCM input
function origin_new = fcn(origin,CoM,DCM)
%#codegen
origin_new=zeros(3,3);
for i=1:3
    origin_new(i,:)=(DCM*origin(i,:)'+CoM)';
end

== matlab function Full_system_3DOF/image_effect ==
  data: OS_mu input; F_body_images output; OS_xyz input; OS_mu_fc input; fc_xyz input; origin input; tau_body_images output; U_images output; CoM input
function [F_body_images,tau_body_images,U_images]=image_effect(OS_mu,OS_xyz,...
    OS_mu_fc,fc_xyz,origin,CoM)
%#codegen

%F_body_images is the total force on the body due to mobile and frozen
% image effects
%tau_body_images is the total torque on the body due to mobile and frozen
% image effects
%frozen_lists and mobile_lists keeps track of the individual mobile and
% frozen image effects
%OS_mu are the magnetic moment dipoles of the permanent magnets on the OS
%OS_xyz are the magnet positions on the OS
%OS_mu_fc are the field cooled magnetic moment dipoles of the permanent
% magnets on the OS
%fc_xyz are the field cooled positions of the permanent magnets on the OS
%origin is an arbitrary point on the superconductor surface that I have
% chosen to be the center of the superconductor disk surface

%F_body_sum and tau_body_sum is to keep track of the communative effort of
%all frozen and mobile images on magnet i, correlating to row i
F_body_sum=zeros(size(OS_mu,1),3);
tau_body_sum=zeros(size(OS_mu,1),3);
U_fsum=zeros(size(OS_mu,1),1);
U_msum=zeros(size(OS_mu,1),1);
%frozen_lists and mobile_lists goes more in depth than F_body_sum and
%tau_body_sum, storing the individual effect of every frozen and mobile
%image where:
%the first column represents magnet i
%the second column represents magnet j
%third to fifth columns represent force on magnet i due to j's image
%sixth to eighth columns represent torque on magnet i due to j's image
% frozen_lists=zeros(size(OS_mu,1)^2,8,size(origin,1));
% mobile_lists=zeros(size(OS_mu,1)^2,8,size(origin,1));


%% Sum frozen and mobile images across different superconductors and all magnets
for k=1:size(origin,1) %sift through all the superconductors
    %initialize row counter
    row=1;
    for i=1:size(OS_xyz,1) %sift through all the magnets i
        
        mu_mag_i=OS_mu(i,:);
        pos_mag_i=OS_xyz(i,:);
        O=origin(k,:);
        
        for j=1:size(OS_xyz,1) %sift through all the magnets j that generate images
            
            mu_mag_j=OS_mu(j,:);
            pos_mag_j=OS_xyz(j,:);
            mu_mag_fc=OS_mu_fc(j,:);
            pos_fc=fc_xyz(j,:);

            %find the contribution of each field cooled image on all the
            %permanent magnets
            effect='frozen';
            [F,tau,U]=calculate_Ftau(mu_mag_i,mu_mag_j,mu_mag_fc,...
                pos_mag_i,pos_mag_j,pos_fc,O,effect);

            F_body_sum(i,:)=F_body_sum(i,:)+F;
            tau_body_sum(i,:)=tau_body_sum(i,:)+tau+cross(pos_mag_i-CoM',F);
            U_fsum(i)=U_fsum(i)+U;
            %this list is for debugging storing all frozen image effects,
            %first column the magnet, second column the frozen image, 3:5
            %column the force, 6:8 the torque
%             frozen_lists(row,1,k)=i;
%             frozen_lists(row,2,k)=j;
%             frozen_lists(row,3:5,k)=F;
%             frozen_lists(row,6:8,k)=tau;      

            %find the contribution of this magnet's mobile image on
            %the i_th source magnet
            effect='mobile';
            [F,tau,U]=calculate_Ftau(mu_mag_i,mu_mag_j,mu_mag_fc,...
                pos_mag_i,pos_mag_j,pos_fc,O,effect);
            
            F_body_sum(i,:)=F_body_sum(i,:)+F;
            tau_body_sum(i,:)=tau_body_sum(i,:)+tau+cross(pos_mag_i-CoM',F);
            U_msum(i)=U_msum(i)+U;
            %this list is for debugging storing all mobile image effects,
            %first column the magnet, second column the frozen image, 3:5
            %column the force, 6:8 the torque
%             mobile_lists(row,1,k)=i;
%             mobile_lists(row,2,k)=j;
%             mobile_lists(row,3:5,k)=F;
%             mobile_lists(row,6:8,k)=tau;

            row=row+1;
        end
    end
end

%sum columns to get the total force and torque on the body
F_body_images=sum(F_body_sum,1)';
tau_body_images=sum(tau_body_sum,1)';
U_images=[sum(U_fsum) sum(U_msum)];

== matlab function Full_system_3DOF/rigid_body_dynamics_3DOF/body2magfull ==
  data: B_m input; OS_CoM input; OS_mu output; DCM input; OS_xyz output
function [OS_mu,OS_xyz] = body2mag(B_m,OS_CoM,DCM)
%#codegen
tau=(1+sqrt(5))/2;
OS_xyz=[0 1 tau;
    -1 tau 0;
    1 tau 0;
    0 1 -tau;
    0 -1 tau;
    0 -1 -tau;
    1 -tau 0;
    -1 -tau 0;
    tau 0 1;
    tau 0 -1;
    -tau 0 -1;
    -tau 0 1];
%^the coordinate points of an icosahedron
D=20.3/100; %m the diameter of the OS
magd=1.905/100; %m the diameter of the 0.75 inch spherical magnets to use
rM=(D-magd)/2; %m this radius corresponds to the center of the magnets 
%so that the magnets are flush against the OS surface
OS_magmom=zeros(size(OS_xyz));
for i=1:size(OS_xyz,1)
    OS_magmom(i,:)=(DCM*OS_xyz(i,:)'/norm(OS_xyz(i,:)))';
    OS_xyz(i,:)=OS_magmom(i,:)*rM+OS_CoM';
end
%the permeability of free space, mu_0
mu_0=4*pi*10^-7; %N/A^2

%surface strength of the magnetic field of the dipole measured along its
%dipole axis taken from manufacturer's website
% B_m=8815e-4; %Tesla

%distance from the center of the magnet to its surface
d_m=1.905/2/100; %m

%the estimated magnetic dipole moment magnitude for each magnet on the OS
%surface
OS_mu=2*pi*B_m*d_m^3/mu_0*OS_magmom;
